simulink model "boostLeadControl"  (R2013b)
settings: Solver=ode3  SolverMode=SingleTasking  StartTime=0.0  StopTime=10  RelTol=1e-3
values from neighbouring files (symbols this model uses):
  Ts = 0.01    [Control2lab1.mat]
libraries: arduino_io_lib x4
settings Model: ExtModeTrigDuration=2  Creator=gcampa  LastModifiedBy=richard.hill
settings DataIOCC: SignalLoggingSaveFormat=ModelDataLogs
settings OptimizationCC: OptimizeModelRefInitCode=on  LifeSpan=1
settings DebuggingCC: SolverPrmCheckMsg=none  MultiTaskDSMMsg=warning  MultiTaskCondExecSysMsg=none  StrictBusMsg=None
settings HardwareCC: ProdBitPerInt=16  ProdBitPerPointer=8  ProdIntDivRoundTo=Zero  ProdEndianess=LittleEndian  ProdWordSize=8  ProdHWDeviceType=Atmel->AVR
settings RTWCC: SystemTargetFile=realtime.tlc  GenerateMakefile=off  TemplateMakefile=realtime.tmf  Description=Run on Target Hardware  RTWVerbose=off  ProcessScript=realtime_make_rtw_hook  IncludeERTFirstTime=on
settings STFCustomTargetCC: TargetLibSuffix=.a  CodeReplacementLibrary=None  GenerateSampleERTMain=on  ERTCustomFileBanners=on  SupportNonInlinedSFcns=off  SupportVariableSizeSignals=on  MATLABClassNameForMDSCustomization=Simulink.SoftwareTarget.ERTCustomization  GRTInterface=off  SystemTargetFile=realtime.tlc
settings ERTTargetCC: GenerateSampleERTMain=on  ParMdlRefBuildCompliant=off  CompOptLevelCompliant=off  ConcurrentExecutionCompliant=off  CombineOutputUpdateFcns=off  ERTFirstTimeCompliant=off  SupportContinuousTime=on  SupportVariableSizeSignals=on  ModelStepFunctionPrototypeControlCompliant=off  CPPClassGenCompliant=off  ExtModeTransport=3  ExtModeMexFile=ext_serial_win32_comm  ExtModeMexArgs=0 1 9600  InlinedParameterPlacement=NonHierarchical  ERTSrcFileBannerTemplate=realtime_code_template.cgt  ERTHdrFileBannerTemplate=realtime_code_template.cgt  ERTDataSrcFileTemplate=realtime_code_template.cgt  ERTDataHdrFileTemplate=realtime_code_template.cgt  ERTCustomFileTemplate=realtime_file_process.tlc

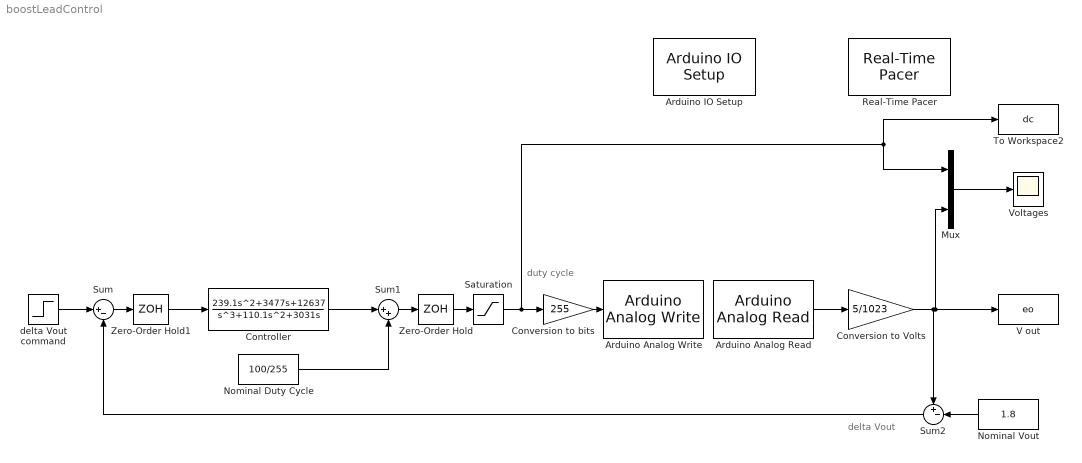
== system boostLeadControl ==
  note: delta Vout
  note: duty cycle
  Arduino Analog Read : arduino_io_lib/Arduino Analog Read  arduinoVar=Temporary arduino variable: Arduino1  arduinoPin=0  T=Ts
  Arduino Analog Write : arduino_io_lib/Arduino Analog Write  arduinoVar=Temporary arduino variable: Arduino1  arduinoPin=9  T=-1
  Arduino IO Setup : arduino_io_lib/Arduino IO Setup  Priority=3  arduinoVar=Temporary arduino variable: Arduino1  workspaceVarName=b  comPort=COM4
  Controller : TransferFcn  Numerator=[239.1 3477 12637]  Denominator=[1 110.1 3031 0]
  Conversion to Volts : Gain  Gain=5/1023
  Conversion to bits : Gain  Gain=255
  Mux : Mux  Inputs=2
  Nominal Duty Cycle : Constant  Value=100/255
  Nominal Vout : Constant  Value=1.8
  Real-Time Pacer : arduino_io_lib/Real-Time Pacer  simTimePerRealTime=1
  Saturation : Saturate  UpperLimit=1  LowerLimit=0
  Sum : Sum  Inputs=|+-
  Sum1 : Sum  Inputs=|++
  Sum2 : Sum  Inputs=+-|
  To Workspace2 : ToWorkspace  VariableName=dc  SampleTime=-1  SaveFormat=Timeseries
  V out : ToWorkspace  VariableName=eo  SampleTime=-1  SaveFormat=Timeseries
  Voltages : Scope
  Zero-Order Hold : ZeroOrderHold  SampleTime=Ts
  Zero-Order Hold1 : ZeroOrderHold  SampleTime=Ts
  delta Vout command : Step  Time=3  SampleTime=Ts
  wires:
  Arduino Analog Read/1 -> Conversion to Volts/1
  Mux/1 -> Voltages/1
  Conversion to Volts/1 -> V out/1, Mux/2, Sum2/1
  delta Vout command/1 -> Sum/1
  Saturation/1 -> Mux/1, To Workspace2/1, Conversion to bits/1
  Conversion to bits/1 -> Arduino Analog Write/1
  Sum1/1 -> Zero-Order Hold/1
  Nominal Duty Cycle/1 -> Sum1/2
  Sum2/1 -> Sum/2
  Nominal Vout/1 -> Sum2/2
  Zero-Order Hold/1 -> Saturation/1
  Zero-Order Hold1/1 -> Controller/1
  Sum/1 -> Zero-Order Hold1/1
  Controller/1 -> Sum1/1
